simulink model "Controller_HIL"  (R2024a)
settings: Solver=FixedStepDiscrete  StartTime=0.0  StopTime=inf  FixedStep=ts_controller  RelTol=1e-3
InitFcn:
  | mbd_s32k_consistency_checks(bdroot(gcs));
undefined symbols (not defined in the file): Battery, BMS_Controller_State, Charging_State, currentFactor, CV_Gain, DiscIntNeverNeededParam, I_cc, LQFP, MaxCellVoltThrsld, noCurrent, Ns_Module, NumModules, OverCellVoltageLimit, SOCInit, SRE, ts_controller, ts_system, UnderCellVoltageLimit, voltThreshold
libraries: mbd_s32k1xx_ec_toolbox x104, etargetslib x95, mbd_bcc_ec_toolbox x30, hdlsllib x11, simulink x6, sharedTrackingLibrary x2
(part 3 of 4)

== system Controller_HIL/CAN Rx/RX_FIFO_Complete_Event/Temperature/Action_Rx_0x2 ==
  Data : Inport
  Action Port : ActionPort  ActionPortLabel=case [ 1033 ]:
  Byte Unpack : etargetslib/Byte Unpack  dimensions={[1] [1]}  datatypes={'single', 'single'}  byteAlign=1
      settings: LibrarySourceBlock=embeddedtargetslib/Host Communication/Byte Unpack
  FCAN_Receive_FIFO : mbd_s32k1xx_ec_toolbox/Communication Blocks/CAN Blocks/FCAN_Receive  can_instance=0  can_mode=Non-blocking  can_timeout_ms=0  can_mb_idx=0  can_mb_init=Once  show_id_input=off  can_extended_id=off  can_is_remote=off  can_id=0x7FF  can_msg_mask=0  show_adv_opts=on  can_use_rxfifo=on  can_fd_enable=off
  Outport : Outport
  Outport1 : Outport  Port=2
  wires:
  Data/1 -> Byte Unpack/1
  Byte Unpack/2 -> Outport1/1
  Byte Unpack/1 -> Outport/1

== system Controller_HIL/CAN Rx/RX_FIFO_Complete_Event/Temperature/Action_Rx_0x20 ==
  Data : Inport
  Action Port : ActionPort  ActionPortLabel=case [ 1063 ]:
  Byte Unpack : etargetslib/Byte Unpack  dimensions={[1] [1]}  datatypes={'single', 'single'}  byteAlign=1
      settings: LibrarySourceBlock=embeddedtargetslib/Host Communication/Byte Unpack
  FCAN_Receive_FIFO : mbd_s32k1xx_ec_toolbox/Communication Blocks/CAN Blocks/FCAN_Receive  can_instance=0  can_mode=Non-blocking  can_timeout_ms=0  can_mb_idx=0  can_mb_init=Once  show_id_input=off  can_extended_id=off  can_is_remote=off  can_id=0x7FF  can_msg_mask=0  show_adv_opts=on  can_use_rxfifo=on  can_fd_enable=off
  Outport : Outport
  Outport1 : Outport  Port=2
  wires:
  Data/1 -> Byte Unpack/1
  Byte Unpack/2 -> Outport1/1
  Byte Unpack/1 -> Outport/1

== system Controller_HIL/CAN Rx/RX_FIFO_Complete_Event/Temperature/Action_Rx_0x21 ==
  Data : Inport
  Action Port : ActionPort  ActionPortLabel=case [ 1064 ]:
  Byte Unpack : etargetslib/Byte Unpack  dimensions={[1] [1]}  datatypes={'single', 'single'}  byteAlign=1
      settings: LibrarySourceBlock=embeddedtargetslib/Host Communication/Byte Unpack
  FCAN_Receive_FIFO : mbd_s32k1xx_ec_toolbox/Communication Blocks/CAN Blocks/FCAN_Receive  can_instance=0  can_mode=Non-blocking  can_timeout_ms=0  can_mb_idx=0  can_mb_init=Once  show_id_input=off  can_extended_id=off  can_is_remote=off  can_id=0x7FF  can_msg_mask=0  show_adv_opts=on  can_use_rxfifo=on  can_fd_enable=off
  Outport : Outport
  Outport1 : Outport  Port=2
  wires:
  Byte Unpack/1 -> Outport/1
  Byte Unpack/2 -> Outport1/1
  Data/1 -> Byte Unpack/1

== system Controller_HIL/CAN Rx/RX_FIFO_Complete_Event/Temperature/Action_Rx_0x22 ==
  Data : Inport
  Action Port : ActionPort  ActionPortLabel=case [ 1065 ]:
  Byte Unpack : etargetslib/Byte Unpack  dimensions={[1] [1]}  datatypes={'single', 'single'}  byteAlign=1
      settings: LibrarySourceBlock=embeddedtargetslib/Host Communication/Byte Unpack
  FCAN_Receive_FIFO : mbd_s32k1xx_ec_toolbox/Communication Blocks/CAN Blocks/FCAN_Receive  can_instance=0  can_mode=Non-blocking  can_timeout_ms=0  can_mb_idx=0  can_mb_init=Once  show_id_input=off  can_extended_id=off  can_is_remote=off  can_id=0x7FF  can_msg_mask=0  show_adv_opts=on  can_use_rxfifo=on  can_fd_enable=off
  Outport : Outport
  Outport1 : Outport  Port=2
  wires:
  Data/1 -> Byte Unpack/1
  Byte Unpack/1 -> Outport/1
  Byte Unpack/2 -> Outport1/1

== system Controller_HIL/CAN Rx/RX_FIFO_Complete_Event/Temperature/Action_Rx_0x23 ==
  Data : Inport
  Action Port : ActionPort  ActionPortLabel=case [ 1072 ]:
  Byte Unpack : etargetslib/Byte Unpack  dimensions={[1] [1]}  datatypes={'single', 'single'}  byteAlign=1
      settings: LibrarySourceBlock=embeddedtargetslib/Host Communication/Byte Unpack
  FCAN_Receive_FIFO : mbd_s32k1xx_ec_toolbox/Communication Blocks/CAN Blocks/FCAN_Receive  can_instance=0  can_mode=Non-blocking  can_timeout_ms=0  can_mb_idx=0  can_mb_init=Once  show_id_input=off  can_extended_id=off  can_is_remote=off  can_id=0x7FF  can_msg_mask=0  show_adv_opts=on  can_use_rxfifo=on  can_fd_enable=off
  Outport : Outport
  Outport1 : Outport  Port=2
  wires:
  Data/1 -> Byte Unpack/1
  Byte Unpack/2 -> Outport1/1
  Byte Unpack/1 -> Outport/1

== system Controller_HIL/CAN Rx/RX_FIFO_Complete_Event/Temperature/Action_Rx_0x24 ==
  Data : Inport
  Action Port : ActionPort  ActionPortLabel=case [ 1073 ]:
  Byte Unpack : etargetslib/Byte Unpack  dimensions={[1] [1]}  datatypes={'single', 'single'}  byteAlign=1
      settings: LibrarySourceBlock=embeddedtargetslib/Host Communication/Byte Unpack
  FCAN_Receive_FIFO : mbd_s32k1xx_ec_toolbox/Communication Blocks/CAN Blocks/FCAN_Receive  can_instance=0  can_mode=Non-blocking  can_timeout_ms=0  can_mb_idx=0  can_mb_init=Once  show_id_input=off  can_extended_id=off  can_is_remote=off  can_id=0x7FF  can_msg_mask=0  show_adv_opts=on  can_use_rxfifo=on  can_fd_enable=off
  Outport : Outport
  Outport1 : Outport  Port=2
  wires:
  Byte Unpack/1 -> Outport/1
  Byte Unpack/2 -> Outport1/1
  Data/1 -> Byte Unpack/1

== system Controller_HIL/CAN Rx/RX_FIFO_Complete_Event/Temperature/Action_Rx_0x25 ==
  Data : Inport
  Action Port : ActionPort  ActionPortLabel=case [ 1074 ]:
  Byte Unpack : etargetslib/Byte Unpack  dimensions={[1] [1]}  datatypes={'single', 'single'}  byteAlign=1
      settings: LibrarySourceBlock=embeddedtargetslib/Host Communication/Byte Unpack
  FCAN_Receive_FIFO : mbd_s32k1xx_ec_toolbox/Communication Blocks/CAN Blocks/FCAN_Receive  can_instance=0  can_mode=Non-blocking  can_timeout_ms=0  can_mb_idx=0  can_mb_init=Once  show_id_input=off  can_extended_id=off  can_is_remote=off  can_id=0x7FF  can_msg_mask=0  show_adv_opts=on  can_use_rxfifo=on  can_fd_enable=off
  Outport : Outport
  Outport1 : Outport  Port=2
  wires:
  Data/1 -> Byte Unpack/1
  Byte Unpack/1 -> Outport/1
  Byte Unpack/2 -> Outport1/1

== system Controller_HIL/CAN Rx/RX_FIFO_Complete_Event/Temperature/Action_Rx_0x26 ==
  Data : Inport
  Action Port : ActionPort  ActionPortLabel=case [ 1075 ]:
  Byte Unpack : etargetslib/Byte Unpack  dimensions={[1] [1]}  datatypes={'single', 'single'}  byteAlign=1
      settings: LibrarySourceBlock=embeddedtargetslib/Host Communication/Byte Unpack
  FCAN_Receive_FIFO : mbd_s32k1xx_ec_toolbox/Communication Blocks/CAN Blocks/FCAN_Receive  can_instance=0  can_mode=Non-blocking  can_timeout_ms=0  can_mb_idx=0  can_mb_init=Once  show_id_input=off  can_extended_id=off  can_is_remote=off  can_id=0x7FF  can_msg_mask=0  show_adv_opts=on  can_use_rxfifo=on  can_fd_enable=off
  Outport : Outport
  Outport1 : Outport  Port=2
  wires:
  Data/1 -> Byte Unpack/1
  Byte Unpack/2 -> Outport1/1
  Byte Unpack/1 -> Outport/1

== system Controller_HIL/CAN Rx/RX_FIFO_Complete_Event/Temperature/Action_Rx_0x27 ==
  Data : Inport
  Action Port : ActionPort  ActionPortLabel=case [ 1076 ]:
  Byte Unpack : etargetslib/Byte Unpack  dimensions={[1] [1]}  datatypes={'single', 'single'}  byteAlign=1
      settings: LibrarySourceBlock=embeddedtargetslib/Host Communication/Byte Unpack
  FCAN_Receive_FIFO : mbd_s32k1xx_ec_toolbox/Communication Blocks/CAN Blocks/FCAN_Receive  can_instance=0  can_mode=Non-blocking  can_timeout_ms=0  can_mb_idx=0  can_mb_init=Once  show_id_input=off  can_extended_id=off  can_is_remote=off  can_id=0x7FF  can_msg_mask=0  show_adv_opts=on  can_use_rxfifo=on  can_fd_enable=off
  Outport : Outport
  Outport1 : Outport  Port=2
  wires:
  Byte Unpack/1 -> Outport/1
  Byte Unpack/2 -> Outport1/1
  Data/1 -> Byte Unpack/1

== system Controller_HIL/CAN Rx/RX_FIFO_Complete_Event/Temperature/Action_Rx_0x28 ==
  Data : Inport
  Action Port : ActionPort  ActionPortLabel=case [ 1077 ]:
  Byte Unpack : etargetslib/Byte Unpack  dimensions={[1] [1]}  datatypes={'single', 'single'}  byteAlign=1
      settings: LibrarySourceBlock=embeddedtargetslib/Host Communication/Byte Unpack
  FCAN_Receive_FIFO : mbd_s32k1xx_ec_toolbox/Communication Blocks/CAN Blocks/FCAN_Receive  can_instance=0  can_mode=Non-blocking  can_timeout_ms=0  can_mb_idx=0  can_mb_init=Once  show_id_input=off  can_extended_id=off  can_is_remote=off  can_id=0x7FF  can_msg_mask=0  show_adv_opts=on  can_use_rxfifo=on  can_fd_enable=off
  Outport : Outport
  Outport1 : Outport  Port=2
  wires:
  Data/1 -> Byte Unpack/1
  Byte Unpack/1 -> Outport/1
  Byte Unpack/2 -> Outport1/1

== system Controller_HIL/CAN Rx/RX_FIFO_Complete_Event/Temperature/Action_Rx_0x29 ==
  Data : Inport
  Action Port : ActionPort  ActionPortLabel=case [ 1078 ]:
  Byte Unpack : etargetslib/Byte Unpack  dimensions={[1] [1]}  datatypes={'single', 'single'}  byteAlign=1
      settings: LibrarySourceBlock=embeddedtargetslib/Host Communication/Byte Unpack
  FCAN_Receive_FIFO : mbd_s32k1xx_ec_toolbox/Communication Blocks/CAN Blocks/FCAN_Receive  can_instance=0  can_mode=Non-blocking  can_timeout_ms=0  can_mb_idx=0  can_mb_init=Once  show_id_input=off  can_extended_id=off  can_is_remote=off  can_id=0x7FF  can_msg_mask=0  show_adv_opts=on  can_use_rxfifo=on  can_fd_enable=off
  Outport : Outport
  Outport1 : Outport  Port=2
  wires:
  Data/1 -> Byte Unpack/1
  Byte Unpack/2 -> Outport1/1
  Byte Unpack/1 -> Outport/1

== system Controller_HIL/CAN Rx/RX_FIFO_Complete_Event/Temperature/Action_Rx_0x3 ==
  Data : Inport
  Action Port : ActionPort  ActionPortLabel=case [ 1040 ]:
  Byte Unpack : etargetslib/Byte Unpack  dimensions={[1] [1]}  datatypes={'single', 'single'}  byteAlign=1
      settings: LibrarySourceBlock=embeddedtargetslib/Host Communication/Byte Unpack
  FCAN_Receive_FIFO : mbd_s32k1xx_ec_toolbox/Communication Blocks/CAN Blocks/FCAN_Receive  can_instance=0  can_mode=Non-blocking  can_timeout_ms=0  can_mb_idx=0  can_mb_init=Once  show_id_input=off  can_extended_id=off  can_is_remote=off  can_id=0x7FF  can_msg_mask=0  show_adv_opts=on  can_use_rxfifo=on  can_fd_enable=off
  Outport : Outport
  Outport1 : Outport  Port=2
  wires:
  Byte Unpack/1 -> Outport/1
  Byte Unpack/2 -> Outport1/1
  Data/1 -> Byte Unpack/1

== system Controller_HIL/CAN Rx/RX_FIFO_Complete_Event/Temperature/Action_Rx_0x30 ==
  Data : Inport
  Action Port : ActionPort  ActionPortLabel=case [ 1079 ]:
  Byte Unpack : etargetslib/Byte Unpack  dimensions={[1] [1]}  datatypes={'single', 'single'}  byteAlign=1
      settings: LibrarySourceBlock=embeddedtargetslib/Host Communication/Byte Unpack
  FCAN_Receive_FIFO : mbd_s32k1xx_ec_toolbox/Communication Blocks/CAN Blocks/FCAN_Receive  can_instance=0  can_mode=Non-blocking  can_timeout_ms=0  can_mb_idx=0  can_mb_init=Once  show_id_input=off  can_extended_id=off  can_is_remote=off  can_id=0x7FF  can_msg_mask=0  show_adv_opts=on  can_use_rxfifo=on  can_fd_enable=off
  Outport : Outport
  Outport1 : Outport  Port=2
  wires:
  Byte Unpack/1 -> Outport/1
  Byte Unpack/2 -> Outport1/1
  Data/1 -> Byte Unpack/1

== system Controller_HIL/CAN Rx/RX_FIFO_Complete_Event/Temperature/Action_Rx_0x31 ==
  Data : Inport
  Action Port : ActionPort  ActionPortLabel=case [ 1080 ]:
  Byte Unpack : etargetslib/Byte Unpack  dimensions={[1] [1]}  datatypes={'single', 'single'}  byteAlign=1
      settings: LibrarySourceBlock=embeddedtargetslib/Host Communication/Byte Unpack
  FCAN_Receive_FIFO : mbd_s32k1xx_ec_toolbox/Communication Blocks/CAN Blocks/FCAN_Receive  can_instance=0  can_mode=Non-blocking  can_timeout_ms=0  can_mb_idx=0  can_mb_init=Once  show_id_input=off  can_extended_id=off  can_is_remote=off  can_id=0x7FF  can_msg_mask=0  show_adv_opts=on  can_use_rxfifo=on  can_fd_enable=off
  Outport : Outport
  Outport1 : Outport  Port=2
  wires:
  Data/1 -> Byte Unpack/1
  Byte Unpack/1 -> Outport/1
  Byte Unpack/2 -> Outport1/1

== system Controller_HIL/CAN Rx/RX_FIFO_Complete_Event/Temperature/Action_Rx_0x32 ==
  Data : Inport
  Action Port : ActionPort  ActionPortLabel=case [ 1081 ]:
  Byte Unpack : etargetslib/Byte Unpack  dimensions={[1] [1]}  datatypes={'single', 'single'}  byteAlign=1
      settings: LibrarySourceBlock=embeddedtargetslib/Host Communication/Byte Unpack
  FCAN_Receive_FIFO : mbd_s32k1xx_ec_toolbox/Communication Blocks/CAN Blocks/FCAN_Receive  can_instance=0  can_mode=Non-blocking  can_timeout_ms=0  can_mb_idx=0  can_mb_init=Once  show_id_input=off  can_extended_id=off  can_is_remote=off  can_id=0x7FF  can_msg_mask=0  show_adv_opts=on  can_use_rxfifo=on  can_fd_enable=off
  Outport : Outport
  Outport1 : Outport  Port=2
  wires:
  Data/1 -> Byte Unpack/1
  Byte Unpack/2 -> Outport1/1
  Byte Unpack/1 -> Outport/1

== system Controller_HIL/CAN Rx/RX_FIFO_Complete_Event/Temperature/Action_Rx_0x33 ==
  Data : Inport
  Action Port : ActionPort  ActionPortLabel=case [ 1088 ]:
  Byte Unpack : etargetslib/Byte Unpack  dimensions={[1] [1]}  datatypes={'single', 'single'}  byteAlign=1
      settings: LibrarySourceBlock=embeddedtargetslib/Host Communication/Byte Unpack
  FCAN_Receive_FIFO : mbd_s32k1xx_ec_toolbox/Communication Blocks/CAN Blocks/FCAN_Receive  can_instance=0  can_mode=Non-blocking  can_timeout_ms=0  can_mb_idx=0  can_mb_init=Once  show_id_input=off  can_extended_id=off  can_is_remote=off  can_id=0x7FF  can_msg_mask=0  show_adv_opts=on  can_use_rxfifo=on  can_fd_enable=off
  Outport : Outport
  Outport1 : Outport  Port=2
  wires:
  Byte Unpack/1 -> Outport/1
  Byte Unpack/2 -> Outport1/1
  Data/1 -> Byte Unpack/1

== system Controller_HIL/CAN Rx/RX_FIFO_Complete_Event/Temperature/Action_Rx_0x34 ==
  Data : Inport
  Action Port : ActionPort  ActionPortLabel=case [ 1089 ]:
  Byte Unpack : etargetslib/Byte Unpack  dimensions={[1] [1]}  datatypes={'single', 'single'}  byteAlign=1
      settings: LibrarySourceBlock=embeddedtargetslib/Host Communication/Byte Unpack
  FCAN_Receive_FIFO : mbd_s32k1xx_ec_toolbox/Communication Blocks/CAN Blocks/FCAN_Receive  can_instance=0  can_mode=Non-blocking  can_timeout_ms=0  can_mb_idx=0  can_mb_init=Once  show_id_input=off  can_extended_id=off  can_is_remote=off  can_id=0x7FF  can_msg_mask=0  show_adv_opts=on  can_use_rxfifo=on  can_fd_enable=off
  Outport : Outport
  Outport1 : Outport  Port=2
  wires:
  Data/1 -> Byte Unpack/1
  Byte Unpack/1 -> Outport/1
  Byte Unpack/2 -> Outport1/1

== system Controller_HIL/CAN Rx/RX_FIFO_Complete_Event/Temperature/Action_Rx_0x35 ==
  Data : Inport
  Action Port : ActionPort  ActionPortLabel=case [ 1090 ]:
  Byte Unpack : etargetslib/Byte Unpack  dimensions={[1] [1]}  datatypes={'single', 'single'}  byteAlign=1
      settings: LibrarySourceBlock=embeddedtargetslib/Host Communication/Byte Unpack
  FCAN_Receive_FIFO : mbd_s32k1xx_ec_toolbox/Communication Blocks/CAN Blocks/FCAN_Receive  can_instance=0  can_mode=Non-blocking  can_timeout_ms=0  can_mb_idx=0  can_mb_init=Once  show_id_input=off  can_extended_id=off  can_is_remote=off  can_id=0x7FF  can_msg_mask=0  show_adv_opts=on  can_use_rxfifo=on  can_fd_enable=off
  Outport : Outport
  Outport1 : Outport  Port=2
  wires:
  Data/1 -> Byte Unpack/1
  Byte Unpack/2 -> Outport1/1
  Byte Unpack/1 -> Outport/1

== system Controller_HIL/CAN Rx/RX_FIFO_Complete_Event/Temperature/Action_Rx_0x36 ==
  Data : Inport
  Action Port : ActionPort  ActionPortLabel=case [ 1091 ]:
  Byte Unpack : etargetslib/Byte Unpack  dimensions={[1] [1]}  datatypes={'single', 'single'}  byteAlign=1
      settings: LibrarySourceBlock=embeddedtargetslib/Host Communication/Byte Unpack
  FCAN_Receive_FIFO : mbd_s32k1xx_ec_toolbox/Communication Blocks/CAN Blocks/FCAN_Receive  can_instance=0  can_mode=Non-blocking  can_timeout_ms=0  can_mb_idx=0  can_mb_init=Once  show_id_input=off  can_extended_id=off  can_is_remote=off  can_id=0x7FF  can_msg_mask=0  show_adv_opts=on  can_use_rxfifo=on  can_fd_enable=off
  Outport : Outport
  Outport1 : Outport  Port=2
  wires:
  Byte Unpack/1 -> Outport/1
  Byte Unpack/2 -> Outport1/1
  Data/1 -> Byte Unpack/1

== system Controller_HIL/CAN Rx/RX_FIFO_Complete_Event/Temperature/Action_Rx_0x37 ==
  Data : Inport
  Action Port : ActionPort  ActionPortLabel=case [ 1092 ]:
  Byte Unpack : etargetslib/Byte Unpack  dimensions={[1] [1]}  datatypes={'single', 'single'}  byteAlign=1
      settings: LibrarySourceBlock=embeddedtargetslib/Host Communication/Byte Unpack
  FCAN_Receive_FIFO : mbd_s32k1xx_ec_toolbox/Communication Blocks/CAN Blocks/FCAN_Receive  can_instance=0  can_mode=Non-blocking  can_timeout_ms=0  can_mb_idx=0  can_mb_init=Once  show_id_input=off  can_extended_id=off  can_is_remote=off  can_id=0x7FF  can_msg_mask=0  show_adv_opts=on  can_use_rxfifo=on  can_fd_enable=off
  Outport : Outport
  Outport1 : Outport  Port=2
  wires:
  Data/1 -> Byte Unpack/1
  Byte Unpack/2 -> Outport1/1
  Byte Unpack/1 -> Outport/1

== system Controller_HIL/CAN Rx/RX_FIFO_Complete_Event/Temperature/Action_Rx_0x38 ==
  Data : Inport
  Action Port : ActionPort  ActionPortLabel=case [ 1093 ]:
  Byte Unpack : etargetslib/Byte Unpack  dimensions={[1] [1]}  datatypes={'single', 'single'}  byteAlign=1
      settings: LibrarySourceBlock=embeddedtargetslib/Host Communication/Byte Unpack
  FCAN_Receive_FIFO : mbd_s32k1xx_ec_toolbox/Communication Blocks/CAN Blocks/FCAN_Receive  can_instance=0  can_mode=Non-blocking  can_timeout_ms=0  can_mb_idx=0  can_mb_init=Once  show_id_input=off  can_extended_id=off  can_is_remote=off  can_id=0x7FF  can_msg_mask=0  show_adv_opts=on  can_use_rxfifo=on  can_fd_enable=off
  Outport : Outport
  Outport1 : Outport  Port=2
  wires:
  Byte Unpack/1 -> Outport/1
  Byte Unpack/2 -> Outport1/1
  Data/1 -> Byte Unpack/1

== system Controller_HIL/CAN Rx/RX_FIFO_Complete_Event/Temperature/Action_Rx_0x39 ==
  Data : Inport
  Action Port : ActionPort  ActionPortLabel=case [ 1094 ]:
  Byte Unpack : etargetslib/Byte Unpack  dimensions={[1] [1]}  datatypes={'single', 'single'}  byteAlign=1
      settings: LibrarySourceBlock=embeddedtargetslib/Host Communication/Byte Unpack
  FCAN_Receive_FIFO : mbd_s32k1xx_ec_toolbox/Communication Blocks/CAN Blocks/FCAN_Receive  can_instance=0  can_mode=Non-blocking  can_timeout_ms=0  can_mb_idx=0  can_mb_init=Once  show_id_input=off  can_extended_id=off  can_is_remote=off  can_id=0x7FF  can_msg_mask=0  show_adv_opts=on  can_use_rxfifo=on  can_fd_enable=off
  Outport : Outport
  Outport1 : Outport  Port=2
  wires:
  Byte Unpack/1 -> Outport/1
  Byte Unpack/2 -> Outport1/1
  Data/1 -> Byte Unpack/1

== system Controller_HIL/CAN Rx/RX_FIFO_Complete_Event/Temperature/Action_Rx_0x4 ==
  Data : Inport
  Action Port : ActionPort  ActionPortLabel=case [ 1041 ]:
  Byte Unpack : etargetslib/Byte Unpack  dimensions={[1] [1]}  datatypes={'single', 'single'}  byteAlign=1
      settings: LibrarySourceBlock=embeddedtargetslib/Host Communication/Byte Unpack
  FCAN_Receive_FIFO : mbd_s32k1xx_ec_toolbox/Communication Blocks/CAN Blocks/FCAN_Receive  can_instance=0  can_mode=Non-blocking  can_timeout_ms=0  can_mb_idx=0  can_mb_init=Once  show_id_input=off  can_extended_id=off  can_is_remote=off  can_id=0x7FF  can_msg_mask=0  show_adv_opts=on  can_use_rxfifo=on  can_fd_enable=off
  Outport : Outport
  Outport1 : Outport  Port=2
  wires:
  Data/1 -> Byte Unpack/1
  Byte Unpack/1 -> Outport/1
  Byte Unpack/2 -> Outport1/1

== system Controller_HIL/CAN Rx/RX_FIFO_Complete_Event/Temperature/Action_Rx_0x40 ==
  Data : Inport
  Action Port : ActionPort  ActionPortLabel=case [ 1095 ]:
  Byte Unpack : etargetslib/Byte Unpack  dimensions={[1] [1]}  datatypes={'single', 'single'}  byteAlign=1
      settings: LibrarySourceBlock=embeddedtargetslib/Host Communication/Byte Unpack
  FCAN_Receive_FIFO : mbd_s32k1xx_ec_toolbox/Communication Blocks/CAN Blocks/FCAN_Receive  can_instance=0  can_mode=Non-blocking  can_timeout_ms=0  can_mb_idx=0  can_mb_init=Once  show_id_input=off  can_extended_id=off  can_is_remote=off  can_id=0x7FF  can_msg_mask=0  show_adv_opts=on  can_use_rxfifo=on  can_fd_enable=off
  Outport : Outport
  Outport1 : Outport  Port=2
  wires:
  Data/1 -> Byte Unpack/1
  Byte Unpack/1 -> Outport/1
  Byte Unpack/2 -> Outport1/1

== system Controller_HIL/CAN Rx/RX_FIFO_Complete_Event/Temperature/Action_Rx_0x401 ==
  Data : Inport
  Action Port : ActionPort  ActionPortLabel=case [ 1025 ]:
  Byte Unpack : etargetslib/Byte Unpack  dimensions={[1] [1]}  datatypes={'single', 'uint32'}  byteAlign=1
      settings: LibrarySourceBlock=embeddedtargetslib/Host Communication/Byte Unpack
  FCAN_Receive_FIFO : mbd_s32k1xx_ec_toolbox/Communication Blocks/CAN Blocks/FCAN_Receive  can_instance=0  can_mode=Non-blocking  can_timeout_ms=0  can_mb_idx=0  can_mb_init=Once  show_id_input=off  can_extended_id=off  can_is_remote=off  can_id=0x7FF  can_msg_mask=0  show_adv_opts=on  can_use_rxfifo=on  can_fd_enable=off
  Outport : Outport
  Outport1 : Outport  Port=2
  wires:
  Data/1 -> Byte Unpack/1
  Byte Unpack/1 -> Outport/1
  Byte Unpack/2 -> Outport1/1

== system Controller_HIL/CAN Rx/RX_FIFO_Complete_Event/Temperature/Action_Rx_0x402 ==
  Data : Inport
  Action Port : ActionPort  ActionPortLabel=case [ 1026 ]:
  Byte Unpack : etargetslib/Byte Unpack  dimensions={[1] [1]}  datatypes={'single', 'single'}  byteAlign=1
      settings: LibrarySourceBlock=embeddedtargetslib/Host Communication/Byte Unpack
  FCAN_Receive_FIFO : mbd_s32k1xx_ec_toolbox/Communication Blocks/CAN Blocks/FCAN_Receive  can_instance=0  can_mode=Non-blocking  can_timeout_ms=0  can_mb_idx=0  can_mb_init=Once  show_id_input=off  can_extended_id=off  can_is_remote=off  can_id=0x7FF  can_msg_mask=0  show_adv_opts=on  can_use_rxfifo=on  can_fd_enable=off
  Outport : Outport
  Outport1 : Outport  Port=2
  wires:
  Data/1 -> Byte Unpack/1
  Byte Unpack/1 -> Outport/1
  Byte Unpack/2 -> Outport1/1

== system Controller_HIL/CAN Rx/RX_FIFO_Complete_Event/Temperature/Action_Rx_0x403 ==
  Data : Inport
  Action Port : ActionPort  ActionPortLabel=case [ 1027 ]:
  Byte Unpack : etargetslib/Byte Unpack  dimensions={[1] [1]}  datatypes={'single', 'single'}  byteAlign=1
      settings: LibrarySourceBlock=embeddedtargetslib/Host Communication/Byte Unpack
  FCAN_Receive_FIFO : mbd_s32k1xx_ec_toolbox/Communication Blocks/CAN Blocks/FCAN_Receive  can_instance=0  can_mode=Non-blocking  can_timeout_ms=0  can_mb_idx=0  can_mb_init=Once  show_id_input=off  can_extended_id=off  can_is_remote=off  can_id=0x7FF  can_msg_mask=0  show_adv_opts=on  can_use_rxfifo=on  can_fd_enable=off
  Outport : Outport
  Outport1 : Outport  Port=2
  wires:
  Data/1 -> Byte Unpack/1
  Byte Unpack/2 -> Outport1/1
  Byte Unpack/1 -> Outport/1

== system Controller_HIL/CAN Rx/RX_FIFO_Complete_Event/Temperature/Action_Rx_0x404 ==
  Data : Inport
  Action Port : ActionPort  ActionPortLabel=case [ 1028 ]:
  Byte Unpack : etargetslib/Byte Unpack  dimensions={[1] [1]}  datatypes={'single', 'single'}  byteAlign=1
      settings: LibrarySourceBlock=embeddedtargetslib/Host Communication/Byte Unpack
  FCAN_Receive_FIFO : mbd_s32k1xx_ec_toolbox/Communication Blocks/CAN Blocks/FCAN_Receive  can_instance=0  can_mode=Non-blocking  can_timeout_ms=0  can_mb_idx=0  can_mb_init=Once  show_id_input=off  can_extended_id=off  can_is_remote=off  can_id=0x7FF  can_msg_mask=0  show_adv_opts=on  can_use_rxfifo=on  can_fd_enable=off
  Outport : Outport
  Outport1 : Outport  Port=2
  wires:
  Byte Unpack/1 -> Outport/1
  Byte Unpack/2 -> Outport1/1
  Data/1 -> Byte Unpack/1

== system Controller_HIL/CAN Rx/RX_FIFO_Complete_Event/Temperature/Action_Rx_0x405 ==
  Data : Inport
  Action Port : ActionPort  ActionPortLabel=case [ 1029 ]:
  Byte Unpack : etargetslib/Byte Unpack  dimensions={[1] [1]}  datatypes={'single', 'single'}  byteAlign=1
      settings: LibrarySourceBlock=embeddedtargetslib/Host Communication/Byte Unpack
  FCAN_Receive_FIFO : mbd_s32k1xx_ec_toolbox/Communication Blocks/CAN Blocks/FCAN_Receive  can_instance=0  can_mode=Non-blocking  can_timeout_ms=0  can_mb_idx=0  can_mb_init=Once  show_id_input=off  can_extended_id=off  can_is_remote=off  can_id=0x7FF  can_msg_mask=0  show_adv_opts=on  can_use_rxfifo=on  can_fd_enable=off
  Outport : Outport
  Outport1 : Outport  Port=2
  wires:
  Data/1 -> Byte Unpack/1
  Byte Unpack/1 -> Outport/1
  Byte Unpack/2 -> Outport1/1

== system Controller_HIL/CAN Rx/RX_FIFO_Complete_Event/Temperature/Action_Rx_0x406 ==
  Data : Inport
  Action Port : ActionPort  ActionPortLabel=case [ 1030 ]:
  Byte Unpack : etargetslib/Byte Unpack  dimensions={[1] [1]}  datatypes={'single', 'single'}  byteAlign=1
      settings: LibrarySourceBlock=embeddedtargetslib/Host Communication/Byte Unpack
  FCAN_Receive_FIFO : mbd_s32k1xx_ec_toolbox/Communication Blocks/CAN Blocks/FCAN_Receive  can_instance=0  can_mode=Non-blocking  can_timeout_ms=0  can_mb_idx=0  can_mb_init=Once  show_id_input=off  can_extended_id=off  can_is_remote=off  can_id=0x7FF  can_msg_mask=0  show_adv_opts=on  can_use_rxfifo=on  can_fd_enable=off
  Outport : Outport
  Outport1 : Outport  Port=2
  wires:
  Data/1 -> Byte Unpack/1
  Byte Unpack/2 -> Outport1/1
  Byte Unpack/1 -> Outport/1

== system Controller_HIL/CAN Rx/RX_FIFO_Complete_Event/Temperature/Action_Rx_0x407 ==
  Data : Inport
  Action Port : ActionPort  ActionPortLabel=case [ 1031 ]:
  Byte Unpack : etargetslib/Byte Unpack  dimensions={[1] [1]}  datatypes={'single', 'single'}  byteAlign=1
      settings: LibrarySourceBlock=embeddedtargetslib/Host Communication/Byte Unpack
  FCAN_Receive_FIFO : mbd_s32k1xx_ec_toolbox/Communication Blocks/CAN Blocks/FCAN_Receive  can_instance=0  can_mode=Non-blocking  can_timeout_ms=0  can_mb_idx=0  can_mb_init=Once  show_id_input=off  can_extended_id=off  can_is_remote=off  can_id=0x7FF  can_msg_mask=0  show_adv_opts=on  can_use_rxfifo=on  can_fd_enable=off
  Outport : Outport
  Outport1 : Outport  Port=2
  wires:
  Byte Unpack/1 -> Outport/1
  Byte Unpack/2 -> Outport1/1
  Data/1 -> Byte Unpack/1

== system Controller_HIL/CAN Rx/RX_FIFO_Complete_Event/Temperature/Action_Rx_0x41 ==
  Data : Inport
  Action Port : ActionPort  ActionPortLabel=case [ 1096 ]:
  Byte Unpack : etargetslib/Byte Unpack  dimensions={[1] [1]}  datatypes={'single', 'single'}  byteAlign=1
      settings: LibrarySourceBlock=embeddedtargetslib/Host Communication/Byte Unpack
  FCAN_Receive_FIFO : mbd_s32k1xx_ec_toolbox/Communication Blocks/CAN Blocks/FCAN_Receive  can_instance=0  can_mode=Non-blocking  can_timeout_ms=0  can_mb_idx=0  can_mb_init=Once  show_id_input=off  can_extended_id=off  can_is_remote=off  can_id=0x7FF  can_msg_mask=0  show_adv_opts=on  can_use_rxfifo=on  can_fd_enable=off
  Outport : Outport
  Outport1 : Outport  Port=2
  wires:
  Data/1 -> Byte Unpack/1
  Byte Unpack/2 -> Outport1/1
  Byte Unpack/1 -> Outport/1

== system Controller_HIL/CAN Rx/RX_FIFO_Complete_Event/Temperature/Action_Rx_0x42 ==
  Data : Inport
  Action Port : ActionPort  ActionPortLabel=case [ 1097 ]:
  Byte Unpack : etargetslib/Byte Unpack  dimensions={[1] [1]}  datatypes={'single', 'single'}  byteAlign=1
      settings: LibrarySourceBlock=embeddedtargetslib/Host Communication/Byte Unpack
  FCAN_Receive_FIFO : mbd_s32k1xx_ec_toolbox/Communication Blocks/CAN Blocks/FCAN_Receive  can_instance=0  can_mode=Non-blocking  can_timeout_ms=0  can_mb_idx=0  can_mb_init=Once  show_id_input=off  can_extended_id=off  can_is_remote=off  can_id=0x7FF  can_msg_mask=0  show_adv_opts=on  can_use_rxfifo=on  can_fd_enable=off
  Outport : Outport
  Outport1 : Outport  Port=2
  wires:
  Byte Unpack/1 -> Outport/1
  Byte Unpack/2 -> Outport1/1
  Data/1 -> Byte Unpack/1

== system Controller_HIL/CAN Rx/RX_FIFO_Complete_Event/Temperature/Action_Rx_0x43 ==
  Data : Inport
  Action Port : ActionPort  ActionPortLabel=case [ 1104 ]:
  Byte Unpack : etargetslib/Byte Unpack  dimensions={[1] [1]}  datatypes={'single', 'single'}  byteAlign=1
      settings: LibrarySourceBlock=embeddedtargetslib/Host Communication/Byte Unpack
  FCAN_Receive_FIFO : mbd_s32k1xx_ec_toolbox/Communication Blocks/CAN Blocks/FCAN_Receive  can_instance=0  can_mode=Non-blocking  can_timeout_ms=0  can_mb_idx=0  can_mb_init=Once  show_id_input=off  can_extended_id=off  can_is_remote=off  can_id=0x7FF  can_msg_mask=0  show_adv_opts=on  can_use_rxfifo=on  can_fd_enable=off
  Outport : Outport
  Outport1 : Outport  Port=2
  wires:
  Data/1 -> Byte Unpack/1
  Byte Unpack/2 -> Outport1/1
  Byte Unpack/1 -> Outport/1

== system Controller_HIL/CAN Rx/RX_FIFO_Complete_Event/Temperature/Action_Rx_0x44 ==
  Data : Inport
  Action Port : ActionPort  ActionPortLabel=case [ 1105 ]:
  Byte Unpack : etargetslib/Byte Unpack  dimensions={[1] [1]}  datatypes={'single', 'single'}  byteAlign=1
      settings: LibrarySourceBlock=embeddedtargetslib/Host Communication/Byte Unpack
  FCAN_Receive_FIFO : mbd_s32k1xx_ec_toolbox/Communication Blocks/CAN Blocks/FCAN_Receive  can_instance=0  can_mode=Non-blocking  can_timeout_ms=0  can_mb_idx=0  can_mb_init=Once  show_id_input=off  can_extended_id=off  can_is_remote=off  can_id=0x7FF  can_msg_mask=0  show_adv_opts=on  can_use_rxfifo=on  can_fd_enable=off
  Outport : Outport
  Outport1 : Outport  Port=2
  wires:
  Byte Unpack/1 -> Outport/1
  Byte Unpack/2 -> Outport1/1
  Data/1 -> Byte Unpack/1

== system Controller_HIL/CAN Rx/RX_FIFO_Complete_Event/Temperature/Action_Rx_0x5 ==
  Data : Inport
  Action Port : ActionPort  ActionPortLabel=case [ 1042 ]:
  Byte Unpack : etargetslib/Byte Unpack  dimensions={[1] [1]}  datatypes={'single', 'single'}  byteAlign=1
      settings: LibrarySourceBlock=embeddedtargetslib/Host Communication/Byte Unpack
  FCAN_Receive_FIFO : mbd_s32k1xx_ec_toolbox/Communication Blocks/CAN Blocks/FCAN_Receive  can_instance=0  can_mode=Non-blocking  can_timeout_ms=0  can_mb_idx=0  can_mb_init=Once  show_id_input=off  can_extended_id=off  can_is_remote=off  can_id=0x7FF  can_msg_mask=0  show_adv_opts=on  can_use_rxfifo=on  can_fd_enable=off
  Outport : Outport
  Outport1 : Outport  Port=2
  wires:
  Data/1 -> Byte Unpack/1
  Byte Unpack/2 -> Outport1/1
  Byte Unpack/1 -> Outport/1

== system Controller_HIL/CAN Rx/RX_FIFO_Complete_Event/Temperature/Action_Rx_0x6 ==
  Data : Inport
  Action Port : ActionPort  ActionPortLabel=case [ 1043 ]:
  Byte Unpack : etargetslib/Byte Unpack  dimensions={[1] [1]}  datatypes={'single', 'single'}  byteAlign=1
      settings: LibrarySourceBlock=embeddedtargetslib/Host Communication/Byte Unpack
  FCAN_Receive_FIFO : mbd_s32k1xx_ec_toolbox/Communication Blocks/CAN Blocks/FCAN_Receive  can_instance=0  can_mode=Non-blocking  can_timeout_ms=0  can_mb_idx=0  can_mb_init=Once  show_id_input=off  can_extended_id=off  can_is_remote=off  can_id=0x7FF  can_msg_mask=0  show_adv_opts=on  can_use_rxfifo=on  can_fd_enable=off
  Outport : Outport
  Outport1 : Outport  Port=2
  wires:
  Byte Unpack/1 -> Outport/1
  Byte Unpack/2 -> Outport1/1
  Data/1 -> Byte Unpack/1

== system Controller_HIL/CAN Rx/RX_FIFO_Complete_Event/Temperature/Action_Rx_0x7 ==
  Data : Inport
  Action Port : ActionPort  ActionPortLabel=case [ 1044 ]:
  Byte Unpack : etargetslib/Byte Unpack  dimensions={[1] [1]}  datatypes={'single', 'single'}  byteAlign=1
      settings: LibrarySourceBlock=embeddedtargetslib/Host Communication/Byte Unpack
  FCAN_Receive_FIFO : mbd_s32k1xx_ec_toolbox/Communication Blocks/CAN Blocks/FCAN_Receive  can_instance=0  can_mode=Non-blocking  can_timeout_ms=0  can_mb_idx=0  can_mb_init=Once  show_id_input=off  can_extended_id=off  can_is_remote=off  can_id=0x7FF  can_msg_mask=0  show_adv_opts=on  can_use_rxfifo=on  can_fd_enable=off
  Outport : Outport
  Outport1 : Outport  Port=2
  wires:
  Data/1 -> Byte Unpack/1
  Byte Unpack/1 -> Outport/1
  Byte Unpack/2 -> Outport1/1

== system Controller_HIL/CAN Rx/RX_FIFO_Complete_Event/Temperature/Action_Rx_0x8 ==
  Data : Inport
  Action Port : ActionPort  ActionPortLabel=case [ 1045 ]:
  Byte Unpack : etargetslib/Byte Unpack  dimensions={[1] [1]}  datatypes={'single', 'single'}  byteAlign=1
      settings: LibrarySourceBlock=embeddedtargetslib/Host Communication/Byte Unpack
  FCAN_Receive_FIFO : mbd_s32k1xx_ec_toolbox/Communication Blocks/CAN Blocks/FCAN_Receive  can_instance=0  can_mode=Non-blocking  can_timeout_ms=0  can_mb_idx=0  can_mb_init=Once  show_id_input=off  can_extended_id=off  can_is_remote=off  can_id=0x7FF  can_msg_mask=0  show_adv_opts=on  can_use_rxfifo=on  can_fd_enable=off
  Outport : Outport
  Outport1 : Outport  Port=2
  wires:
  Data/1 -> Byte Unpack/1
  Byte Unpack/2 -> Outport1/1
  Byte Unpack/1 -> Outport/1

== system Controller_HIL/CAN Rx/RX_FIFO_Complete_Event/Temperature/Action_Rx_0x9 ==
  Data : Inport
  Action Port : ActionPort  ActionPortLabel=case [ 1046 ]:
  Byte Unpack : etargetslib/Byte Unpack  dimensions={[1] [1]}  datatypes={'single', 'single'}  byteAlign=1
      settings: LibrarySourceBlock=embeddedtargetslib/Host Communication/Byte Unpack
  FCAN_Receive_FIFO : mbd_s32k1xx_ec_toolbox/Communication Blocks/CAN Blocks/FCAN_Receive  can_instance=0  can_mode=Non-blocking  can_timeout_ms=0  can_mb_idx=0  can_mb_init=Once  show_id_input=off  can_extended_id=off  can_is_remote=off  can_id=0x7FF  can_msg_mask=0  show_adv_opts=on  can_use_rxfifo=on  can_fd_enable=off
  Outport : Outport
  Outport1 : Outport  Port=2
  wires:
  Byte Unpack/1 -> Outport/1
  Byte Unpack/2 -> Outport1/1
  Data/1 -> Byte Unpack/1

== system Controller_HIL/CAN Rx/RX_FIFO_Complete_Event/Voltage/Action_Rx_0x1 ==
  Data : Inport
  Action Port : ActionPort  ActionPortLabel=case [ 1112 ]:
  Byte Unpack : etargetslib/Byte Unpack  dimensions={[1] [1]}  datatypes={'single', 'single'}  byteAlign=1
      settings: LibrarySourceBlock=embeddedtargetslib/Host Communication/Byte Unpack
  FCAN_Receive_FIFO : mbd_s32k1xx_ec_toolbox/Communication Blocks/CAN Blocks/FCAN_Receive  can_instance=0  can_mode=Non-blocking  can_timeout_ms=0  can_mb_idx=0  can_mb_init=Once  show_id_input=off  can_extended_id=off  can_is_remote=off  can_id=0x7FF  can_msg_mask=0  show_adv_opts=on  can_use_rxfifo=on  can_fd_enable=off
  Outport : Outport
  Outport1 : Outport  Port=2
  wires:
  Data/1 -> Byte Unpack/1
  Byte Unpack/1 -> Outport/1
  Byte Unpack/2 -> Outport1/1

== system Controller_HIL/CAN Rx/RX_FIFO_Complete_Event/Voltage/Action_Rx_0x10 ==
  Data : Inport
  Action Port : ActionPort  ActionPortLabel=case [ 1127 ]:
  Byte Unpack : etargetslib/Byte Unpack  dimensions={[1] [1]}  datatypes={'single', 'single'}  byteAlign=1
      settings: LibrarySourceBlock=embeddedtargetslib/Host Communication/Byte Unpack
  FCAN_Receive_FIFO : mbd_s32k1xx_ec_toolbox/Communication Blocks/CAN Blocks/FCAN_Receive  can_instance=0  can_mode=Non-blocking  can_timeout_ms=0  can_mb_idx=0  can_mb_init=Once  show_id_input=off  can_extended_id=off  can_is_remote=off  can_id=0x7FF  can_msg_mask=0  show_adv_opts=on  can_use_rxfifo=on  can_fd_enable=off
  Outport : Outport
  Outport1 : Outport  Port=2
  wires:
  Data/1 -> Byte Unpack/1
  Byte Unpack/1 -> Outport/1
  Byte Unpack/2 -> Outport1/1

== system Controller_HIL/CAN Rx/RX_FIFO_Complete_Event/Voltage/Action_Rx_0x11 ==
  Data : Inport
  Action Port : ActionPort  ActionPortLabel=case [ 1128 ]:
  Byte Unpack : etargetslib/Byte Unpack  dimensions={[1] [1]}  datatypes={'single', 'single'}  byteAlign=1
      settings: LibrarySourceBlock=embeddedtargetslib/Host Communication/Byte Unpack
  FCAN_Receive_FIFO : mbd_s32k1xx_ec_toolbox/Communication Blocks/CAN Blocks/FCAN_Receive  can_instance=0  can_mode=Non-blocking  can_timeout_ms=0  can_mb_idx=0  can_mb_init=Once  show_id_input=off  can_extended_id=off  can_is_remote=off  can_id=0x7FF  can_msg_mask=0  show_adv_opts=on  can_use_rxfifo=on  can_fd_enable=off
  Outport : Outport
  Outport1 : Outport  Port=2
  wires:
  Data/1 -> Byte Unpack/1
  Byte Unpack/2 -> Outport1/1
  Byte Unpack/1 -> Outport/1

== system Controller_HIL/CAN Rx/RX_FIFO_Complete_Event/Voltage/Action_Rx_0x12 ==
  Data : Inport
  Action Port : ActionPort  ActionPortLabel=case [ 1129 ]:
  Byte Unpack : etargetslib/Byte Unpack  dimensions={[1] [1]}  datatypes={'single', 'single'}  byteAlign=1
      settings: LibrarySourceBlock=embeddedtargetslib/Host Communication/Byte Unpack
  FCAN_Receive_FIFO : mbd_s32k1xx_ec_toolbox/Communication Blocks/CAN Blocks/FCAN_Receive  can_instance=0  can_mode=Non-blocking  can_timeout_ms=0  can_mb_idx=0  can_mb_init=Once  show_id_input=off  can_extended_id=off  can_is_remote=off  can_id=0x7FF  can_msg_mask=0  show_adv_opts=on  can_use_rxfifo=on  can_fd_enable=off
  Outport : Outport
  Outport1 : Outport  Port=2
  wires:
  Byte Unpack/1 -> Outport/1
  Byte Unpack/2 -> Outport1/1
  Data/1 -> Byte Unpack/1

== system Controller_HIL/CAN Rx/RX_FIFO_Complete_Event/Voltage/Action_Rx_0x13 ==
  Data : Inport
  Action Port : ActionPort  ActionPortLabel=case [ 1136 ]:
  Byte Unpack : etargetslib/Byte Unpack  dimensions={[1] [1]}  datatypes={'single', 'single'}  byteAlign=1
      settings: LibrarySourceBlock=embeddedtargetslib/Host Communication/Byte Unpack
  FCAN_Receive_FIFO : mbd_s32k1xx_ec_toolbox/Communication Blocks/CAN Blocks/FCAN_Receive  can_instance=0  can_mode=Non-blocking  can_timeout_ms=0  can_mb_idx=0  can_mb_init=Once  show_id_input=off  can_extended_id=off  can_is_remote=off  can_id=0x7FF  can_msg_mask=0  show_adv_opts=on  can_use_rxfifo=on  can_fd_enable=off
  Outport : Outport
  Outport1 : Outport  Port=2
  wires:
  Data/1 -> Byte Unpack/1
  Byte Unpack/1 -> Outport/1
  Byte Unpack/2 -> Outport1/1

== system Controller_HIL/CAN Rx/RX_FIFO_Complete_Event/Voltage/Action_Rx_0x14 ==
  Data : Inport
  Action Port : ActionPort  ActionPortLabel=case [ 1137 ]:
  Byte Unpack : etargetslib/Byte Unpack  dimensions={[1] [1]}  datatypes={'single', 'single'}  byteAlign=1
      settings: LibrarySourceBlock=embeddedtargetslib/Host Communication/Byte Unpack
  FCAN_Receive_FIFO : mbd_s32k1xx_ec_toolbox/Communication Blocks/CAN Blocks/FCAN_Receive  can_instance=0  can_mode=Non-blocking  can_timeout_ms=0  can_mb_idx=0  can_mb_init=Once  show_id_input=off  can_extended_id=off  can_is_remote=off  can_id=0x7FF  can_msg_mask=0  show_adv_opts=on  can_use_rxfifo=on  can_fd_enable=off
  Outport : Outport
  Outport1 : Outport  Port=2
  wires:
  Data/1 -> Byte Unpack/1
  Byte Unpack/2 -> Outport1/1
  Byte Unpack/1 -> Outport/1

== system Controller_HIL/CAN Rx/RX_FIFO_Complete_Event/Voltage/Action_Rx_0x15 ==
  Data : Inport
  Action Port : ActionPort  ActionPortLabel=case [ 1138 ]:
  Byte Unpack : etargetslib/Byte Unpack  dimensions={[1] [1]}  datatypes={'single', 'single'}  byteAlign=1
      settings: LibrarySourceBlock=embeddedtargetslib/Host Communication/Byte Unpack
  FCAN_Receive_FIFO : mbd_s32k1xx_ec_toolbox/Communication Blocks/CAN Blocks/FCAN_Receive  can_instance=0  can_mode=Non-blocking  can_timeout_ms=0  can_mb_idx=0  can_mb_init=Once  show_id_input=off  can_extended_id=off  can_is_remote=off  can_id=0x7FF  can_msg_mask=0  show_adv_opts=on  can_use_rxfifo=on  can_fd_enable=off
  Outport : Outport
  Outport1 : Outport  Port=2
  wires:
  Byte Unpack/1 -> Outport/1
  Byte Unpack/2 -> Outport1/1
  Data/1 -> Byte Unpack/1

== system Controller_HIL/CAN Rx/RX_FIFO_Complete_Event/Voltage/Action_Rx_0x16 ==
  Data : Inport
  Action Port : ActionPort  ActionPortLabel=case [ 1139 ]:
  Byte Unpack : etargetslib/Byte Unpack  dimensions={[1] [1]}  datatypes={'single', 'single'}  byteAlign=1
      settings: LibrarySourceBlock=embeddedtargetslib/Host Communication/Byte Unpack
  FCAN_Receive_FIFO : mbd_s32k1xx_ec_toolbox/Communication Blocks/CAN Blocks/FCAN_Receive  can_instance=0  can_mode=Non-blocking  can_timeout_ms=0  can_mb_idx=0  can_mb_init=Once  show_id_input=off  can_extended_id=off  can_is_remote=off  can_id=0x7FF  can_msg_mask=0  show_adv_opts=on  can_use_rxfifo=on  can_fd_enable=off
  Outport : Outport
  Outport1 : Outport  Port=2
  wires:
  Data/1 -> Byte Unpack/1
  Byte Unpack/1 -> Outport/1
  Byte Unpack/2 -> Outport1/1

== system Controller_HIL/CAN Rx/RX_FIFO_Complete_Event/Voltage/Action_Rx_0x17 ==
  Data : Inport
  Action Port : ActionPort  ActionPortLabel=case [ 1140 ]:
  Byte Unpack : etargetslib/Byte Unpack  dimensions={[1] [1]}  datatypes={'single', 'single'}  byteAlign=1
      settings: LibrarySourceBlock=embeddedtargetslib/Host Communication/Byte Unpack
  FCAN_Receive_FIFO : mbd_s32k1xx_ec_toolbox/Communication Blocks/CAN Blocks/FCAN_Receive  can_instance=0  can_mode=Non-blocking  can_timeout_ms=0  can_mb_idx=0  can_mb_init=Once  show_id_input=off  can_extended_id=off  can_is_remote=off  can_id=0x7FF  can_msg_mask=0  show_adv_opts=on  can_use_rxfifo=on  can_fd_enable=off
  Outport : Outport
  Outport1 : Outport  Port=2
  wires:
  Data/1 -> Byte Unpack/1
  Byte Unpack/2 -> Outport1/1
  Byte Unpack/1 -> Outport/1

== system Controller_HIL/CAN Rx/RX_FIFO_Complete_Event/Voltage/Action_Rx_0x18 ==
  Data : Inport
  Action Port : ActionPort  ActionPortLabel=case [ 1141 ]:
  Byte Unpack : etargetslib/Byte Unpack  dimensions={[1] [1]}  datatypes={'single', 'single'}  byteAlign=1
      settings: LibrarySourceBlock=embeddedtargetslib/Host Communication/Byte Unpack
  FCAN_Receive_FIFO : mbd_s32k1xx_ec_toolbox/Communication Blocks/CAN Blocks/FCAN_Receive  can_instance=0  can_mode=Non-blocking  can_timeout_ms=0  can_mb_idx=0  can_mb_init=Once  show_id_input=off  can_extended_id=off  can_is_remote=off  can_id=0x7FF  can_msg_mask=0  show_adv_opts=on  can_use_rxfifo=on  can_fd_enable=off
  Outport : Outport
  Outport1 : Outport  Port=2
  wires:
  Byte Unpack/1 -> Outport/1
  Byte Unpack/2 -> Outport1/1
  Data/1 -> Byte Unpack/1

== system Controller_HIL/CAN Rx/RX_FIFO_Complete_Event/Voltage/Action_Rx_0x19 ==
  Data : Inport
  Action Port : ActionPort  ActionPortLabel=case [ 1142 ]:
  Byte Unpack : etargetslib/Byte Unpack  dimensions={[1] [1]}  datatypes={'single', 'single'}  byteAlign=1
      settings: LibrarySourceBlock=embeddedtargetslib/Host Communication/Byte Unpack
  FCAN_Receive_FIFO : mbd_s32k1xx_ec_toolbox/Communication Blocks/CAN Blocks/FCAN_Receive  can_instance=0  can_mode=Non-blocking  can_timeout_ms=0  can_mb_idx=0  can_mb_init=Once  show_id_input=off  can_extended_id=off  can_is_remote=off  can_id=0x7FF  can_msg_mask=0  show_adv_opts=on  can_use_rxfifo=on  can_fd_enable=off
  Outport : Outport
  Outport1 : Outport  Port=2
  wires:
  Data/1 -> Byte Unpack/1
  Byte Unpack/1 -> Outport/1
  Byte Unpack/2 -> Outport1/1

== system Controller_HIL/CAN Rx/RX_FIFO_Complete_Event/Voltage/Action_Rx_0x2 ==
  Data : Inport
  Action Port : ActionPort  ActionPortLabel=case [ 1113 ]:
  Byte Unpack : etargetslib/Byte Unpack  dimensions={[1] [1]}  datatypes={'single', 'single'}  byteAlign=1
      settings: LibrarySourceBlock=embeddedtargetslib/Host Communication/Byte Unpack
  FCAN_Receive_FIFO : mbd_s32k1xx_ec_toolbox/Communication Blocks/CAN Blocks/FCAN_Receive  can_instance=0  can_mode=Non-blocking  can_timeout_ms=0  can_mb_idx=0  can_mb_init=Once  show_id_input=off  can_extended_id=off  can_is_remote=off  can_id=0x7FF  can_msg_mask=0  show_adv_opts=on  can_use_rxfifo=on  can_fd_enable=off
  Outport : Outport
  Outport1 : Outport  Port=2
  wires:
  Data/1 -> Byte Unpack/1
  Byte Unpack/2 -> Outport1/1
  Byte Unpack/1 -> Outport/1

== system Controller_HIL/CAN Rx/RX_FIFO_Complete_Event/Voltage/Action_Rx_0x20 ==
  Data : Inport
  Action Port : ActionPort  ActionPortLabel=case [ 1143 ]:
  Byte Unpack : etargetslib/Byte Unpack  dimensions={[1] [1]}  datatypes={'single', 'single'}  byteAlign=1
      settings: LibrarySourceBlock=embeddedtargetslib/Host Communication/Byte Unpack
  FCAN_Receive_FIFO : mbd_s32k1xx_ec_toolbox/Communication Blocks/CAN Blocks/FCAN_Receive  can_instance=0  can_mode=Non-blocking  can_timeout_ms=0  can_mb_idx=0  can_mb_init=Once  show_id_input=off  can_extended_id=off  can_is_remote=off  can_id=0x7FF  can_msg_mask=0  show_adv_opts=on  can_use_rxfifo=on  can_fd_enable=off
  Outport : Outport
  Outport1 : Outport  Port=2
  wires:
  Data/1 -> Byte Unpack/1
  Byte Unpack/2 -> Outport1/1
  Byte Unpack/1 -> Outport/1

== system Controller_HIL/CAN Rx/RX_FIFO_Complete_Event/Voltage/Action_Rx_0x21 ==
  Data : Inport
  Action Port : ActionPort  ActionPortLabel=case [ 1144 ]:
  Byte Unpack : etargetslib/Byte Unpack  dimensions={[1] [1]}  datatypes={'single', 'single'}  byteAlign=1
      settings: LibrarySourceBlock=embeddedtargetslib/Host Communication/Byte Unpack
  FCAN_Receive_FIFO : mbd_s32k1xx_ec_toolbox/Communication Blocks/CAN Blocks/FCAN_Receive  can_instance=0  can_mode=Non-blocking  can_timeout_ms=0  can_mb_idx=0  can_mb_init=Once  show_id_input=off  can_extended_id=off  can_is_remote=off  can_id=0x7FF  can_msg_mask=0  show_adv_opts=on  can_use_rxfifo=on  can_fd_enable=off
  Outport : Outport
  Outport1 : Outport  Port=2
  wires:
  Byte Unpack/1 -> Outport/1
  Byte Unpack/2 -> Outport1/1
  Data/1 -> Byte Unpack/1

== system Controller_HIL/CAN Rx/RX_FIFO_Complete_Event/Voltage/Action_Rx_0x22 ==
  Data : Inport
  Action Port : ActionPort  ActionPortLabel=case [ 1145 ]:
  Byte Unpack : etargetslib/Byte Unpack  dimensions={[1] [1]}  datatypes={'single', 'single'}  byteAlign=1
      settings: LibrarySourceBlock=embeddedtargetslib/Host Communication/Byte Unpack
  FCAN_Receive_FIFO : mbd_s32k1xx_ec_toolbox/Communication Blocks/CAN Blocks/FCAN_Receive  can_instance=0  can_mode=Non-blocking  can_timeout_ms=0  can_mb_idx=0  can_mb_init=Once  show_id_input=off  can_extended_id=off  can_is_remote=off  can_id=0x7FF  can_msg_mask=0  show_adv_opts=on  can_use_rxfifo=on  can_fd_enable=off
  Outport : Outport
  Outport1 : Outport  Port=2
  wires:
  Data/1 -> Byte Unpack/1
  Byte Unpack/1 -> Outport/1
  Byte Unpack/2 -> Outport1/1

== system Controller_HIL/CAN Rx/RX_FIFO_Complete_Event/Voltage/Action_Rx_0x23 ==
  Data : Inport
  Action Port : ActionPort  ActionPortLabel=case [ 1152 ]:
  Byte Unpack : etargetslib/Byte Unpack  dimensions={[1] [1]}  datatypes={'single', 'single'}  byteAlign=1
      settings: LibrarySourceBlock=embeddedtargetslib/Host Communication/Byte Unpack
  FCAN_Receive_FIFO : mbd_s32k1xx_ec_toolbox/Communication Blocks/CAN Blocks/FCAN_Receive  can_instance=0  can_mode=Non-blocking  can_timeout_ms=0  can_mb_idx=0  can_mb_init=Once  show_id_input=off  can_extended_id=off  can_is_remote=off  can_id=0x7FF  can_msg_mask=0  show_adv_opts=on  can_use_rxfifo=on  can_fd_enable=off
  Outport : Outport
  Outport1 : Outport  Port=2
  wires:
  Data/1 -> Byte Unpack/1
  Byte Unpack/2 -> Outport1/1
  Byte Unpack/1 -> Outport/1

== system Controller_HIL/CAN Rx/RX_FIFO_Complete_Event/Voltage/Action_Rx_0x24 ==
  Data : Inport
  Action Port : ActionPort  ActionPortLabel=case [ 1153 ]:
  Byte Unpack : etargetslib/Byte Unpack  dimensions={[1] [1]}  datatypes={'single', 'single'}  byteAlign=1
      settings: LibrarySourceBlock=embeddedtargetslib/Host Communication/Byte Unpack
  FCAN_Receive_FIFO : mbd_s32k1xx_ec_toolbox/Communication Blocks/CAN Blocks/FCAN_Receive  can_instance=0  can_mode=Non-blocking  can_timeout_ms=0  can_mb_idx=0  can_mb_init=Once  show_id_input=off  can_extended_id=off  can_is_remote=off  can_id=0x7FF  can_msg_mask=0  show_adv_opts=on  can_use_rxfifo=on  can_fd_enable=off
  Outport : Outport
  Outport1 : Outport  Port=2
  wires:
  Byte Unpack/1 -> Outport/1
  Byte Unpack/2 -> Outport1/1
  Data/1 -> Byte Unpack/1

== system Controller_HIL/CAN Rx/RX_FIFO_Complete_Event/Voltage/Action_Rx_0x25 ==
  Data : Inport
  Action Port : ActionPort  ActionPortLabel=case [ 1154 ]:
  Byte Unpack : etargetslib/Byte Unpack  dimensions={[1] [1]}  datatypes={'single', 'single'}  byteAlign=1
      settings: LibrarySourceBlock=embeddedtargetslib/Host Communication/Byte Unpack
  FCAN_Receive_FIFO : mbd_s32k1xx_ec_toolbox/Communication Blocks/CAN Blocks/FCAN_Receive  can_instance=0  can_mode=Non-blocking  can_timeout_ms=0  can_mb_idx=0  can_mb_init=Once  show_id_input=off  can_extended_id=off  can_is_remote=off  can_id=0x7FF  can_msg_mask=0  show_adv_opts=on  can_use_rxfifo=on  can_fd_enable=off
  Outport : Outport
  Outport1 : Outport  Port=2
  wires:
  Data/1 -> Byte Unpack/1
  Byte Unpack/1 -> Outport/1
  Byte Unpack/2 -> Outport1/1

== system Controller_HIL/CAN Rx/RX_FIFO_Complete_Event/Voltage/Action_Rx_0x26 ==
  Data : Inport
  Action Port : ActionPort  ActionPortLabel=case [ 1155 ]:
  Byte Unpack : etargetslib/Byte Unpack  dimensions={[1] [1]}  datatypes={'single', 'single'}  byteAlign=1
      settings: LibrarySourceBlock=embeddedtargetslib/Host Communication/Byte Unpack
  FCAN_Receive_FIFO : mbd_s32k1xx_ec_toolbox/Communication Blocks/CAN Blocks/FCAN_Receive  can_instance=0  can_mode=Non-blocking  can_timeout_ms=0  can_mb_idx=0  can_mb_init=Once  show_id_input=off  can_extended_id=off  can_is_remote=off  can_id=0x7FF  can_msg_mask=0  show_adv_opts=on  can_use_rxfifo=on  can_fd_enable=off
  Outport : Outport
  Outport1 : Outport  Port=2
  wires:
  Data/1 -> Byte Unpack/1
  Byte Unpack/2 -> Outport1/1
  Byte Unpack/1 -> Outport/1

== system Controller_HIL/CAN Rx/RX_FIFO_Complete_Event/Voltage/Action_Rx_0x27 ==
  Data : Inport
  Action Port : ActionPort  ActionPortLabel=case [ 1156 ]:
  Byte Unpack : etargetslib/Byte Unpack  dimensions={[1] [1]}  datatypes={'single', 'single'}  byteAlign=1
      settings: LibrarySourceBlock=embeddedtargetslib/Host Communication/Byte Unpack
  FCAN_Receive_FIFO : mbd_s32k1xx_ec_toolbox/Communication Blocks/CAN Blocks/FCAN_Receive  can_instance=0  can_mode=Non-blocking  can_timeout_ms=0  can_mb_idx=0  can_mb_init=Once  show_id_input=off  can_extended_id=off  can_is_remote=off  can_id=0x7FF  can_msg_mask=0  show_adv_opts=on  can_use_rxfifo=on  can_fd_enable=off
  Outport : Outport
  Outport1 : Outport  Port=2
  wires:
  Byte Unpack/1 -> Outport/1
  Byte Unpack/2 -> Outport1/1
  Data/1 -> Byte Unpack/1
